simulink model "boost_converter"  (R2022b)
settings: Solver=ode15s  StartTime=0.0  StopTime=2  RelTol=1e-3
libraries: spsCurrentMeasurementLib x2, spsVoltageMeasurementLib x2, spsSeriesRLCBranchLib x2, spsPVArrayLib x1, spsDiodeLib x1, spsMosfetLib x1, sps_lib x1
settings Model: Creator=nisha  LastModifiedBy=nisha

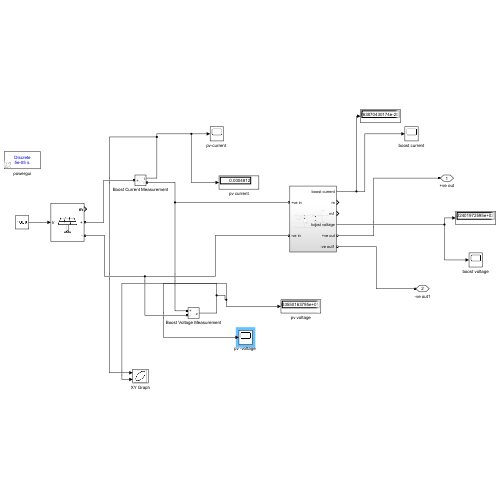
[thumbnail: Simulink's stored preview of the top-level diagram]
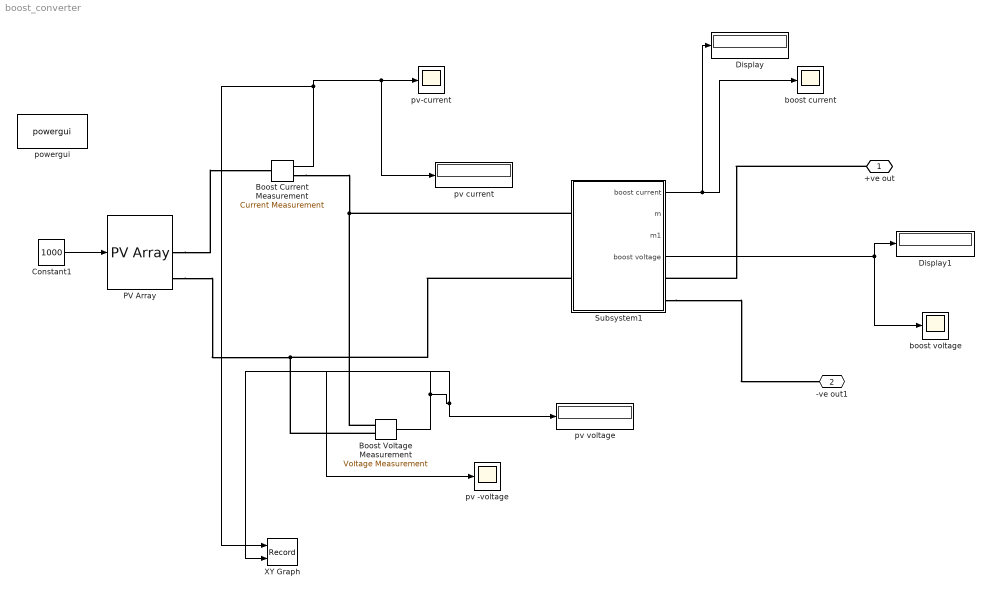
== system boost_converter ==
  Boost Current Measurement : spsCurrentMeasurementLib/Current Measurement  PhasorSimulation=off  OutputType=Complex  PSBequivalent=0
  Boost Voltage Measurement : spsVoltageMeasurementLib/Voltage Measurement  PhasorSimulation=off  OutputType=Complex  PSBequivalent=0
  Constant1 : Constant  Value=1000
  Display : Display
      settings: Format=long_e
  Display1 : Display
      settings: Format=long_e
  PV Array : spsPVArrayLib/PV Array  Npar=1  Nser=1  PlotType=array @ 1000 W/m2 & specified temperatures  S_vec="[ 1000  500  100 ]"  Temp_C_vec="[ 45 25  ]"  ModuleName=User-defined  PlotWhenSelected=off  Pm=213.15  Ncell=60  Voc=96  Isc=7.84  Vm=29  Im=7.35  beta_Voc_pc=-0.36099  alpha_Isc_pc=0.102  beta_Voc=-0.34655  alpha_Isc=0.0079968  IL=10.3099  I0=1.7106e-15  nI=2.3279  Rsh=4.6679  Rs=0.00073371  RobustModel=on  RobustCellTemperature=25  BAL=on  Tc=1e-6  Tfilter=5e-5
  Subsystem1 : Subsystem
  XY Graph : Record  FileSettingsInternal="{\"entries\":[{\"content\":{\"excelSettings\":{\"content\":{},\"type\":\"Streamout.ExcelSettings\"}},\"type\":\"Streamout.FileSettingStorage\",\"uuid\":\"6f3f9a3b-f5d8-4bcf-b94d-3949889a8d48\"}],\"packageUris\":[\"http://schema.mathworks.com/mf0/streamout_blocks/R2020a\"],\"version\":\"1.0\"}"  Layout=[1 1]  SignalsInternal="{\"entries\":[{\"content\":{\"signals\":[{\"content\":{\"blockPath\":[\"boost_converter/XY Graph\"],\"channel\":[],\"dimensions\":[1],\"domain\":\"boost_converter/XY Graph\",\"lineColor\":\"#a2142f\",\"plots\":[1],\"port\":1,\"sid\":[\"\"],\"signalID\":3529,\"signalName\":\"Boost Current Measurement\"},\"type\":\"RecordBlkView.Signal\",\"uuid\":\"c0e0ad29-ebc5-44f6-8a87-7373cebca7da\"},{\"content\":{\"blockPath\":[\"boost_converter/XY Graph\"],\"channel\":[],\"dimensions\":[1],\"domain\":\"boost_converter/XY Graph\",\"lineColor\":\"#139fff\",\"plots\":[1],\"port\":2,\"sid\":[\"\"],\"signalID\":3533,\"signalName\":\"Boost Voltage Measurement\"},\"type\":\"RecordBlkView.Signal\",\"uuid\":\"89dce308-9e66-49ad-9379-be549a4559d5\"}]},\"type\":\"RecordBlkView.InputSignals\",\"uuid\":\"6ba76899-0614-4db0-85c5-08efcea19c2e\"}],\"packageUris\":[\"http://schema.mathworks.com/mf0/streamout_blocks/R2020a\"],\"version\":\"1.0\"}"  VisualizationBindings="{\"xyplotplugin\":{\"info\":[{\"series\":[{\"bindingParametersList\":[{\"parameter\":\"X-Axis\",\"signalID\":3529,\"signalName\":\"Boost Current Measurement\"},{\"parameter\":\"Y-Axis\",\"signalID\":3533,\"signalName\":\"Boost Voltage Measurement\"}],\"seriesID\":56414}],\"subplotID\":1}]}}"  CompatibilityTag=XY
  boost current : Scope
  boost voltage : Scope
  powergui : sps_lib/powergui  Priority=1  SimulationMode=Discrete  SampleTime=5e-5  frequency=60  Iterations=50  frequencyindice=0  Pbase=100e6  ErrMax=1e-4  UnitsV=kV  UnitsW=MW  buscounter=0  FunctionMessages=off  echomessages=off  EnableUseOfTLC=off  CurrentSourceSwitches=off  DisableSnubberDevices=off  DisableRonSwitches=off  DisableVfSwitches=off  DisplayEquations=off  AutomaticDiscreteSolvers=off  SolverType=Tustin/Backward Euler (TBE)  Interpol=off  ExternalGateDelay=off  methode=off  Ts=100  x0status=blocks  SPID=on  SwTol=0  HookPort=off  NonlinearTolerance=1e-4  nMaxIteration=100  ContinueOnMaxIteration=off  RestoreLinks=warning  ResistiveCurrentMeasurement=off  Frange=[0:2:500]  Ylog=off  Xlog=on  ShowGrid=off  save=off  variable=ZData  structure=0  ZoomFFT=off  StartTime=0.0  cycles=1  DisplayStyle=1  fundamental=60  FreqAxis=off  MaxFrequency=1000  frequencyindicesteady=1  RmsSteady=1  display=off
  "pv -voltage " : Scope
  pv current : Display
  pv voltage : Display
      settings: Format=long_e
  "pv-current " : Scope
  +ve out : PMIOPort  Side=Right
  -ve out1 : PMIOPort  Port=2  Side=Right
  wires:
  Subsystem1/1(boost current) -> Display/1, boost current/1
  Subsystem1/4(boost voltage) -> boost voltage/1, Display1/1
  Boost Voltage Measurement/1 -> XY Graph/2, "pv -voltage "/1, pv voltage/1
  Constant1/1 -> PV Array/1
  Boost Current Measurement/1 -> pv current/1, "pv-current "/1, XY Graph/1
  connections:
  Subsystem1/RConn2 -- -ve out1/RConn1
  +ve out/RConn1 -- Subsystem1/RConn1
  Subsystem1/LConn2 -- PV Array/RConn2 -- Boost Voltage Measurement/LConn2
  Subsystem1/LConn1 -- Boost Current Measurement/RConn1 -- Boost Voltage Measurement/LConn1
  PV Array/RConn1 -- Boost Current Measurement/LConn1

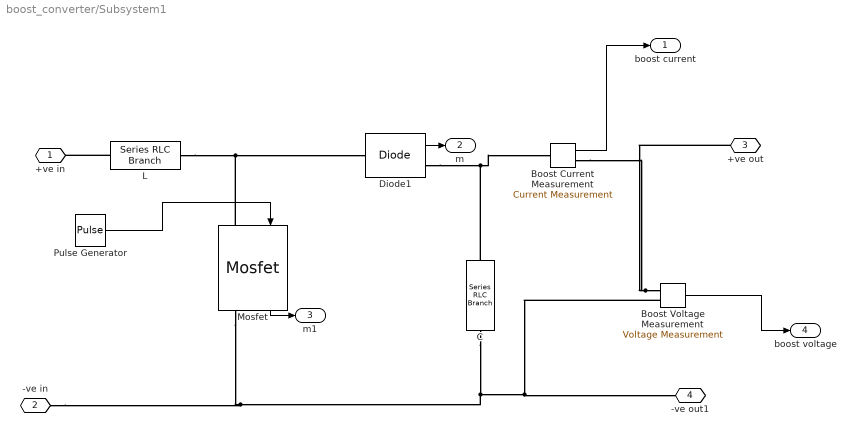
== system boost_converter/Subsystem1 ==
  Boost Current Measurement : spsCurrentMeasurementLib/Current Measurement  PhasorSimulation=off  OutputType=Complex  PSBequivalent=0
  Boost Voltage Measurement : spsVoltageMeasurementLib/Voltage Measurement  PhasorSimulation=off  OutputType=Complex  PSBequivalent=0
  C : spsSeriesRLCBranchLib/Series RLC Branch  LConnTagsString=__new0  RConnTagsString=__new0  BranchType=C  Resistance=1e-3  Inductance=250e-6  SetiL0=off  InitialCurrent=0  Capacitance=1000e-6  Setx0=off  InitialVoltage=0  Measurements=None
  Diode1 : spsDiodeLib/Diode  Ron=0.001  Lon=0  Vf=0.8  IC=0  UseSnubber=0  Rs=500  Cs=250e-9  Measurements=on
  L : spsSeriesRLCBranchLib/Series RLC Branch  LConnTagsString=__new0  RConnTagsString=__new0  BranchType=L  Resistance=1e-3  Inductance=400e-3  SetiL0=off  InitialCurrent=0  Capacitance=1e-6  Setx0=off  InitialVoltage=0  Measurements=None
  Mosfet : spsMosfetLib/Mosfet  Ron=0.1  Lon=0  Rd=0.01  Vfd=0  IC=0  Rs=1e5  Cs=inf  Measurements=on
  Pulse Generator : DiscretePulseGenerator  PulseType=Time based  Period=10  PulseWidth=5
  +ve in : PMIOPort  Side=Left
  -ve in : PMIOPort  Port=2  Side=Left
  +ve out : PMIOPort  Port=3  Side=Right
  -ve out1 : PMIOPort  Port=4  Side=Right
  boost current : Outport
  m : Outport  Port=2
  m1 : Outport  Port=3
  boost voltage : Outport  Port=4
  wires:
  Mosfet/1 -> m1/1
  Boost Current Measurement/1 -> boost current/1
  Pulse Generator/1 -> Mosfet/1
  Boost Voltage Measurement/1 -> boost voltage/1
  Diode1/1 -> m/1
  connections:
  Mosfet/LConn1 -- L/RConn1 -- Diode1/LConn1
  Diode1/RConn1 -- C/LConn1 -- Boost Current Measurement/LConn1
  -ve in/RConn1 -- Mosfet/RConn1 -- C/RConn1 -- Boost Voltage Measurement/LConn2 -- -ve out1/RConn1
  Boost Voltage Measurement/LConn1 -- Boost Current Measurement/RConn1 -- +ve out/RConn1
  L/LConn1 -- +ve in/RConn1
